simulink model "MyobsvOpenLoopSimul"  (R2021b)
settings: Solver=VariableStepAuto  StartTime=0.0  StopTime=200  RelTol=1e-3
undefined symbols (not defined in the file): A, B, C, F, G, L, x0, x_esht_0
settings Model: Creator=tanzc  LastModifiedBy=tanzc
settings DataIOCC: ReturnWorkspaceOutputs=off

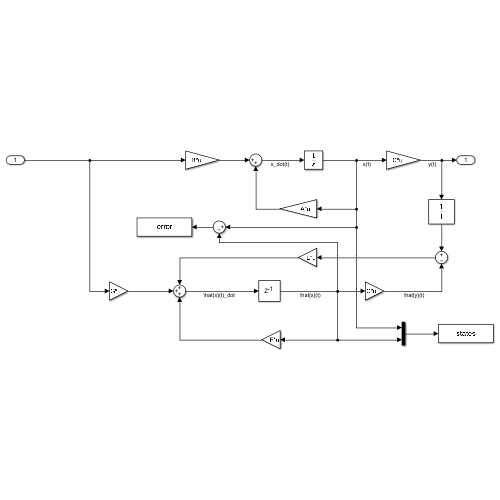
[thumbnail: Simulink's stored preview of the top-level diagram]
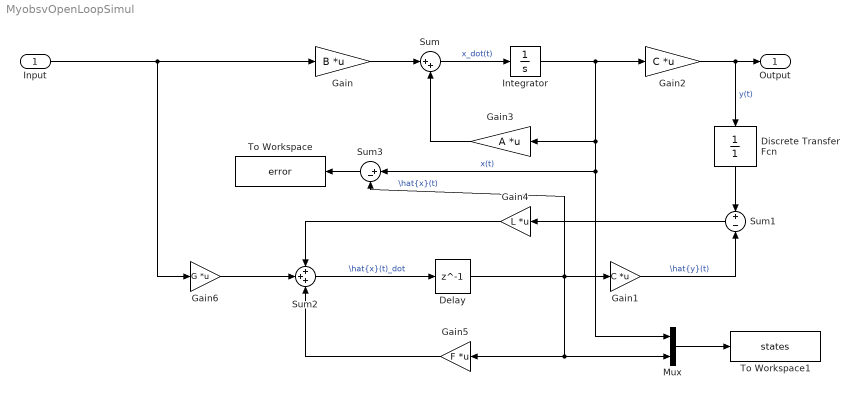
== system MyobsvOpenLoopSimul ==
  Input : Inport  PortDimensions=2
  Delay : Delay  DelayLength=1  InitialCondition=x_esht_0
  Discrete Transfer Fcn : DiscreteTransferFcn  Denominator=1  SampleTime=0.1
  Gain : Gain  Gain=B  Multiplication=Matrix(K*u)
  Gain1 : Gain  Gain=C  Multiplication=Matrix(K*u)
  Gain2 : Gain  Gain=C  Multiplication=Matrix(K*u)
  Gain3 : Gain  Gain=A  Multiplication=Matrix(K*u)
  Gain4 : Gain  Gain=L  Multiplication=Matrix(K*u)
  Gain5 : Gain  Gain=F  Multiplication=Matrix(K*u)
  Gain6 : Gain  Gain=G  Multiplication=Matrix(K*u)
  Integrator : Integrator  InitialCondition=x0
  Mux : Mux  Inputs=2
  Sum : Sum  Inputs=|++
  Sum1 : Sum  Inputs=+-
  Sum2 : Sum  Inputs=+++
  Sum3 : Sum  Inputs=|+-
  To Workspace : ToWorkspace  VariableName=error  SaveFormat=Structure With Time  SampleTime=-1
  To Workspace1 : ToWorkspace  VariableName=states  SaveFormat=Structure With Time  SampleTime=-1
  Output : Outport
  wires:
  Gain/1 -> Sum/1
  Integrator/1 -> Mux/1, Sum3/1, Gain3/1, Gain2/1  "x(t)"
  Sum/1 -> Integrator/1  "x_dot(t)"
  Gain3/1 -> Sum/2
  Gain2/1 -> Discrete Transfer Fcn/1, Output/1  "y(t)"
  Delay/1 -> Mux/2, Gain5/1, Sum3/2, Gain1/1  "\\hat{x}(t)"
  Sum2/1 -> Delay/1  "\\hat{x}(t)_dot"
  Gain1/1 -> Sum1/2  "\\hat{y}(t)"
  Sum1/1 -> Gain4/1
  Gain4/1 -> Sum2/1
  Gain5/1 -> Sum2/3
  Gain6/1 -> Sum2/2
  Input/1 -> Gain6/1, Gain/1
  Sum3/1 -> To Workspace/1
  Mux/1 -> To Workspace1/1
  Discrete Transfer Fcn/1 -> Sum1/1
